simulink model "MDCC"  (R2021b)
settings: Solver=FixedStepDiscrete  StartTime=0.0  StopTime=10.0  FixedStep=0.0001  RelTol=1e-3
model workspace (MATLAB code in the model file):
  | cmdLim = Simulink.Parameter;
  | cmdLim.Value = 15;
  | cmdLim.Description = 'Limit for controlling the maximum surface command angle.';
  | cmdLim.Min = 0;
  | cmdLim.Max = 90;
  | cmdLim.DocUnits = 'deg';
  | 
  | dispGain = Simulink.Parameter;
  | dispGain.Value = 0.75;
  | dispGain.Description = 'Gain applied to the displacement error.';
  | dispGain.Min = 0;
  | dispGain.Max = [];
  | dispGain.DocUnits = 'deg/sec/deg';
  | 
  | dispLim = Simulink.Parameter;
  | dispLim.Value = 30;
  | dispLim.Description = 'Limit for controlling the maximum commanded angle.';
  | dispLim.Min = 0;
  | dispLim.Max = 180;
  | dispLim.DocUnits = 'deg';
  | 
  | intGain = Simulink.Parameter;
  | intGain.Value = 0.5;
  | intGain.Description = 'Gain applied to the integral error.';
  | intGain.Min = 0;
  | intGain.Max = [];
  | intGain.DocUnits = 'deg/sec/deg/sec';
  | 
  | intLim = Simulink.Parameter;
  | intLim.Value = 5;
  | intLim.Description = 'Limit for controlling the maximum commanded angle.';
  | intLim.Min = 0;
  | intLim.Max = 90;
  | intLim.DocUnits = 'deg';
  | 
  | rateGain = Simulink.Parameter;
  | rateGain.Value = 2;
  | rateGain.Description = 'Gain applied to the rate error.';
  | rateGain.Min = 0;
  | rateGain.Max = [];
  | rateGain.DocUnits = 'deg/deg/sec';
  | 
  | rateLim = Simulink.Parameter;
  | rateLim.Value = 6;
  | rateLim.Description = 'Limit for controlling the maximum commanded angle.';
  | rateLim.Min = 0;
  | rateLim.Max = 180;
  | rateLim.DocUnits = 'deg/sec';
  | 
  | hdgGain = Simulink.Parameter;
  | hdgGain.Value = 0.015;
values from neighbouring files (symbols this model uses):
  KfDeadCompen_SetDeltaTime_us = myPackage.Parameter    [DeadCompen.m]
  Ts = 5E-6    (= 5e-06)    [iPMSM_data.m]
  VbDeadComp_SwtUseIsttrDes_flg = myPackage.Parameter    [DeadCompen.m]
  VfDeadCompen_ISttrDdeThdSwt_A = myPackage.Parameter    [DeadCompen.m]
  VfDeadCompen_ISttrIgbtThdSwt_A = myPackage.Parameter    [DeadCompen.m]
  VfDeadCompen_rDdeISttrHi_R = myPackage.Parameter    [DeadCompen.m]
  VfDeadCompen_rDdeISttrLo_R = myPackage.Parameter    [DeadCompen.m]
  VfDeadCompen_rIgbtISttrHi_R = myPackage.Parameter    [DeadCompen.m]
  VfDeadCompen_rIgbtISttrLo_R = myPackage.Parameter    [DeadCompen.m]
  VfDeadCompen_uDdeISttrHi_V = myPackage.Parameter    [DeadCompen.m]
  VfDeadCompen_uDdeISttrLo_V = myPackage.Parameter    [DeadCompen.m]
  VfDeadCompen_uIgbtISttrHi_V = myPackage.Parameter    [DeadCompen.m]
  VfDeadCompen_uIgbtISttrLo_V = myPackage.Parameter    [DeadCompen.m]
undefined symbols (not defined in the file or in its folder): CosTable12bit_Y, GLBCal_GLBCal_Kf_DCLinkOverVolErrThd_V, GLBCal_GLBCal_Kf_DCLinkUnderVolErrThd_V, GLBCal_GLBCal_Kf_EquiLd_NULL, GLBCal_GLBCal_Kf_EquiLq_NULL, GLBCal_GLBCal_Kf_MotorRatedSpeed_rpm, GLBCal_GLBCal_Kf_MotorSpeedHysteresis_Coef, GLBCal_Ke_MotorPolePairsNum_NULL, IoHwAbOpArg_PwmDutyCyclePhU_NULL, IoHwAbOpArg_PwmDutyCyclePhV_NULL, IoHwAbOpArg_PwmDutyCyclePhW_NULL, IoHwAbOpArg_PwmOutputEn, KbMDCC_DeadTimeCompEn_flg, KbMDCC_MCF_flgHarmInIsdqTab11ZR_flg, KbMDCC_MCF_flgHarmInIsdqTab13ZR_flg, KbMDCC_MCF_flgHarmInIsdqTab5ZR_flg, KbMDCC_MCF_flgHarmInIsdqTab7ZR_flg, KbMDCC_MCF_flgHarmInject_flg, KbMDCC_SetEAngleEn_flg, KbMDCC_UdUqFwOmit_flg, KfDeadCompen_CpPeriodTimesT_NULL, KfMDCC_ActiveDischargeIdCurVal_A, KfMDCC_ActiveDischargeIqCurVal_A, KfMDCC_DCLinkVolRate_coef, KfMDCC_DebugEAngleInit_rad, KfMDCC_DebugUalphaVolCmd_V, KfMDCC_DebugUbetaVolCmd_V, KfMDCC_DebugUdCmd_V, KfMDCC_DebugUqCmd_V, KfMDCC_DebugUsCmd_V, KfMDCC_DebugUsRate_V, KfMDCC_IMCResp_NULL, KfMDCC_IMCStab_NULL, KfMDCC_InvParkCpPeriodTimesT_NULL, KfMDCC_MCF_CircAge_NULL, KfMDCC_MCF_flgUse11Harm_flg, KfMDCC_MCF_flgUse13Harm_flg, KfMDCC_MCF_flgUse5Harm_flg, KfMDCC_MCF_flgUse7Harm_flg, KfMDCC_MCF_Harm1113FLParamSpeedThrd_rads, KfMDCC_MCF_Harm57FLParamSpeedThrd_rads, KfMDCC_MCF_HarmcofFltN_NULL, KfMDCC_MCF_HarmCpnAg_NULL, KfMDCC_MCF_HarmfLParaHigh_coef, KfMDCC_MCF_HarmfLParaLow_coef, KfMDCC_MCF_HarmIn1113ZRY_Trq_Nm, KfMDCC_MCF_HarmIn11_SpdLimHigh_rads, KfMDCC_MCF_HarmIn11_SpdLimLow_rads, KfMDCC_MCF_HarmIn11ZRY_Isd_A, KfMDCC_MCF_HarmIn11ZRY_Isq_A, KfMDCC_MCF_HarmIn13_SpdLimHigh_rads, KfMDCC_MCF_HarmIn13_SpdLimLow_rads, KfMDCC_MCF_HarmIn13ZRY_Isd_A, KfMDCC_MCF_HarmIn13ZRY_Isq_A, KfMDCC_MCF_HarmIn57ZRY_Trq_Nm, KfMDCC_MCF_HarmIn5_SpdLimHigh_rads, KfMDCC_MCF_HarmIn5_SpdLimLow_rads, KfMDCC_MCF_HarmIn5ZRY_Isd_A, KfMDCC_MCF_HarmIn5ZRY_Isq_A, KfMDCC_MCF_HarmIn7_SpdLimHigh_rads ... (+47)
libraries: simulink x40, PMSM_Library x3, mcbcontrolslib x1
(part 2 of 8)

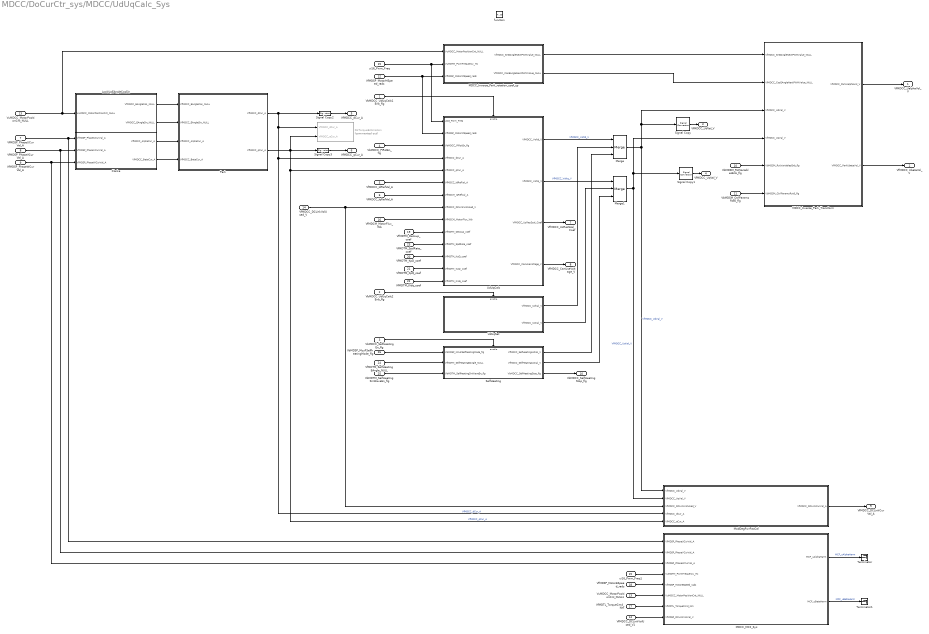
== system MDCC/DoCurCtr_sys/MDCC/UdUqCalc_Sys ==
  VbMDCC_UdUqCalc1Enb_flg : Inport
  VbMDCC_UdUqCalc2Enb_flg : Inport  Port=2
  VbMDCC_SelfHeatingEn_flg : Inport  Port=3
  VbMDCC_PIRstEn_flg : Inport  Port=4
  VfMDCC_IdRefVal_A : Inport  Port=5
  VfMDCC_IqRefVal_A : Inport  Port=6
  VfMDSP_PhaseUCurVal_A : Inport  Port=7
  VfMDSP_PhaseVCurVal_A : Inport  Port=8
  VfMDSP_PhaseWCurVal_A : Inport  Port=9
  VbMDSM_RstVariablesEnb_flg : Inport  Port=10
  VbMDSM_CtrlParamsRst0_flg : Inport  Port=11
  VfMDSP_MotorMSpeed_rads : Inport  Port=12
  VuMDCC_MotorPositionCnt_NULL : Inport  Port=13  OutMin=[0]  OutMax=[4095]
  VfMDCC_DCLinkVolUsed_V : Inport  Port=14
  ui16_Pwm_Freq : Inport  Port=15
  VfMDCM_MotorFlux_Wb : Inport  Port=16
  VfMDTL_TorqueCmd_Nm : Inport  Port=17
  VfMDSP_MotorESpeed_rads : Inport  Port=18
  VfMDTM_Decoup_coef : Inport  Port=19
  VfMDTM_KpD_coef : Inport  Port=20
  VfMDTM_KpQ_coef : Inport  Port=21
  VfMDTM_Kidq_coef : Inport  Port=22
  VfMDTM_SpdRate_coef : Inport  Port=23
  VfMDTM_SelfHeatingEAngle_NULL : Inport  Port=24
  VbMDTM_SelfHeatingSinWaveEn_flg : Inport  Port=25
  VbMDSP_McuFSelfheatingMode_flg : Inport  Port=26
  function : TriggerPort  TriggerType=function-call  VariantControl=Variant  StatesWhenEnabling=reset
      settings: AttributesFormatString=%<StatesWhenEnabling>
  Clarke : Subsystem  TreatAsAtomicUnit=on  RTWFcnName=vPwm_MDCC_Clarke  RTWFileName=MDCC
      settings: RTWSystemCode=Nonreusable function  RTWFcnNameOpts=User specified
  DoTorqueEstimation : Subsystem  Commented=on  TreatAsAtomicUnit=on  RTWFcnName=DoTorqueEstimation  RTWFileName=MDCC
      settings: RTWSystemCode=Nonreusable function  RTWFcnNameOpts=User specified
  LookUpEAngleCosSin : Subsystem  TreatAsAtomicUnit=on  RTWFcnName=vPwm_MDCC_LookUpEAngleCosSin  RTWFileName=MDCC
      settings: RTWSystemCode=Nonreusable function  RTWFcnNameOpts=User specified
  MDCC_Inverse_Park_Transform : Subsystem  TreatAsAtomicUnit=on  RTWFcnName=MDCC_Inverse_Park_Transform  RTWFileName=MDCC
      settings: RTWSystemCode=Nonreusable function  RTWFcnNameOpts=User specified  FunctionWithSeparateData=on
  MDCC_Inverse_Park_rotation_coef_cp : Subsystem  TreatAsAtomicUnit=on  RTWFcnName=MDCC_Inverse_Park_rotation_coef_cp  RTWFileName=MDCC
      settings: RTWSystemCode=Nonreusable function  RTWFcnNameOpts=User specified  FunctionWithSeparateData=on
  MDCC_MCF_Sys : Subsystem
      settings: RTWSystemCode=Nonreusable function  RTWFcnNameOpts=Use subsystem name
  Merge : Merge  Inputs=3
  Merge1 : Merge  Inputs=3
  ModDegPwrFacCal : Subsystem  TreatAsAtomicUnit=on  RTWFcnName=ModDegPwrFacCal  RTWFileName=MDCC
      settings: RTWSystemCode=Nonreusable function  RTWFcnNameOpts=User specified
  Park : Subsystem  TreatAsAtomicUnit=on  RTWFcnName=vPwm_MDCC_Park  RTWFileName=MDCC
      settings: RTWSystemCode=Nonreusable function  RTWFcnNameOpts=User specified
  SelfHeating : Subsystem
  Signal Copy{,1..3} (4 alike) : SignalConversion  OverrideOpt=off
  Terminator : Terminator
  Terminator1 : Terminator
  UdUqCalc : Subsystem  TreatAsAtomicUnit=on  RTWFcnName=MDCC_UdUqCalc
      settings: RTWSystemCode=Nonreusable function  RTWFcnNameOpts=User specified  FunctionWithSeparateData=on
  UdUqSet : Subsystem  RTWFcnName=MDCC_Debug_UdUqSet
      settings: RTWSystemCode=Nonreusable function  RTWFcnNameOpts=User specified
  VfMDCC_DCLinkVolUsed_V1 : InportShadow  Port=14
  VuMDCC_MotorPositionCnt_NULL1 : InportShadow  Port=13  OutMin=[0]  OutMax=[4095]
  ui16_Pwm_Freq1 : InportShadow  Port=15
  VfMDCC_UalphaVol_V : Outport
  VfMDCC_UbetaVol_V : Outport  Port=2
  VfMDCC_UdVal_V : Outport  Port=3
  VfMDCC_UqVal_V : Outport  Port=4
  VfMDCC_dCur_A : Outport  Port=5
  VfMDCC_qCur_A : Outport  Port=6
  VfMDCC_UsResScal_Coef : Outport  Port=7
  VfMDCC_CanUseVoltage_V : Outport  Port=8
  VfMDCC_DCLinkCurVal_A : Outport  Port=9
  VbMDCC_SelfHeatingStop_flg : Outport  Port=10
  wires:
  VfMDCC_IdRefVal_A/1 -> UdUqCalc/6(VfMDCC_IdRefVal_A)
  VfMDCC_IqRefVal_A/1 -> UdUqCalc/7(VfMDCM_IqRefVal_A)
  VfMDSP_MotorMSpeed_rads/1 -> UdUqCalc/2(VfMDSP_MotorMSpeed_rads), MDCC_Inverse_Park_rotation_coef_cp/3(VfMDSP_MotorMSpeed_rads)
  ui16_Pwm_Freq/1 -> UdUqCalc/1(ui16_Pwm_Freq), MDCC_Inverse_Park_rotation_coef_cp/2(VuMDTM_PwmFrequency_Hz)
  VbMDCC_UdUqCalc1Enb_flg/1 -> UdUqCalc/Enable
  VbMDCC_UdUqCalc2Enb_flg/1 -> UdUqSet/Enable
  VbMDSM_RstVariablesEnb_flg/1 -> MDCC_Inverse_Park_Transform/5(VbMDSM_RstVariablesEnb_flg)
  VbMDSM_CtrlParamsRst0_flg/1 -> MDCC_Inverse_Park_Transform/6(VbMDSM_CtrlParamsRst0_flg)
  VuMDCC_MotorPositionCnt_NULL/1 -> MDCC_Inverse_Park_rotation_coef_cp/1(VuMDCC_MotorPositionCnt_NULL), LookUpEAngleCosSin/1(VuMDCC_MotorPositionCnt_NULL)
  LookUpEAngleCosSin/1(VfMDCC_EAngleCos_NULL) -> Park/1(VfMDCC_EAngleCos_NULL)
  Clarke/1(VfMDCC_AlphaCur_A) -> Park/3(VfMDCC_AlphaCur_A)
  Clarke/2(VfMDCC_BetaCur_A) -> Park/4(VfMDCC_BetaCur_A)
  Park/2(VfMDCC_qCur_A) -> DoTorqueEstimation/2(VfMDCC_qCur_A), Signal Copy3/1, ModDegPwrFacCal/5(VfMDCC_qCur_A), UdUqCalc/5(VfMDCC_qCur_A)  "VfMDCC_qCur_A"
  Park/1(VfMDCC_dCur_A) -> ModDegPwrFacCal/4(VfMDCC_dCur_A), UdUqCalc/4(VfMDCC_dCur_A), DoTorqueEstimation/1(VfMDCC_dCur_A), Signal Copy2/1  "VfMDCC_dCur_A"
  LookUpEAngleCosSin/2(VfMDCC_EAngleSin_NULL) -> Park/2(VfMDCC_EAngleSin_NULL)
  VfMDSP_PhaseUCurVal_A/1 -> MDCC_MCF_Sys/1(VfMDSP_PhaseUCurVal_A), Clarke/1(VfMDSP_PhaseUCurVal_A)
  VfMDSP_PhaseVCurVal_A/1 -> MDCC_MCF_Sys/2(VfMDSP_PhaseVCurVal_A), Clarke/2(VfMDSP_PhaseVCurVal_A)
  VfMDSP_PhaseWCurVal_A/1 -> Clarke/3(VfMDSP_PhaseWCurVal_A), MDCC_MCF_Sys/3(VfMDSP_PhaseWCurVal_A)
  MDCC_Inverse_Park_rotation_coef_cp/1(VfMDCC_SinEAngleNextPWMValue_NULL) -> MDCC_Inverse_Park_Transform/1(VfMDCC_SinEAngleNextPWMValue_NULL)
  MDCC_Inverse_Park_rotation_coef_cp/2(VfMDCC_CosEAngleNextPWMValue_NULL) -> MDCC_Inverse_Park_Transform/2(VfMDCC_CosEAngleNextPWMValue_NULL)
  VfMDCC_DCLinkVolUsed_V/1 -> UdUqCalc/8(VfMDCC_DCLinkVolUsed_V), ModDegPwrFacCal/3(VfMDCC_DCLinkVolUsed_V)
  Merge/1 -> ModDegPwrFacCal/1(VfMDCC_UdVal_V), MDCC_Inverse_Park_Transform/3(VfMDCC_UdVal_V), Signal Copy/1  "VfMDCC_UdVal_V"
  Merge1/1 -> MDCC_Inverse_Park_Transform/4(VfMDCC_UqVal_V), Signal Copy1/1, ModDegPwrFacCal/2(VfMDCC_UqVal_V)  "VfMDCC_UqVal_V"
  VfMDCM_MotorFlux_Wb/1 -> UdUqCalc/9(VfMDCM_MotorFlux_Wb)
  UdUqCalc/3(VfMDCC_UsResScal_Coef) -> VfMDCC_UsResScal_Coef/1
  UdUqCalc/4(VfMDCC_CanUseVoltage_V) -> VfMDCC_CanUseVoltage_V/1
  VbMDCC_PIRstEn_flg/1 -> UdUqCalc/3(VbMDCC_PIRstEn_flg)
  Signal Copy/1 -> VfMDCC_UdVal_V/1
  Signal Copy1/1 -> VfMDCC_UqVal_V/1
  UdUqCalc/1(VfMDCC_Voltd_V) -> Merge/1  "VfMDCC_Voltd_V"
  UdUqSet/1(VfMDCC_UdVal_V) -> Merge/2
  UdUqCalc/2(VfMDCC_Voltq_V) -> Merge1/1  "VfMDCC_Voltq_V"
  UdUqSet/2(VfMDCC_UqVal_V) -> Merge1/2
  VfMDSP_MotorESpeed_rads/1 -> MDCC_MCF_Sys/5(VfMDSP_MotorESpeed_rads)
  VfMDTL_TorqueCmd_Nm/1 -> MDCC_MCF_Sys/7(VfMDTL_TorqueCmd_Nm)
  ui16_Pwm_Freq1/1 -> MDCC_MCF_Sys/4(VuMDTM_PwmFrequency_Hz)
  VuMDCC_MotorPositionCnt_NULL1/1 -> MDCC_MCF_Sys/6(VuMDCC_MotorPositionCnt_NULL)
  VfMDCC_DCLinkVolUsed_V1/1 -> MDCC_MCF_Sys/8(VfMDSP_DCLinkVolVal_V)
  MDCC_Inverse_Park_Transform/1(VfMDCC_ParkUalphaVol_V) -> VfMDCC_UalphaVol_V/1
  MDCC_Inverse_Park_Transform/2(VfMDCC_ParkUbetaVol_V) -> VfMDCC_UbetaVol_V/1
  ModDegPwrFacCal/1(VfMDCC_DCLinkCurVal_A) -> VfMDCC_DCLinkCurVal_A/1
  VfMDTM_SpdRate_coef/1 -> UdUqCalc/11(VfMDTM_SpdRate_coef)
  VfMDTM_KpD_coef/1 -> UdUqCalc/12(VfMDTM_KpD_coef)
  VfMDTM_Kidq_coef/1 -> UdUqCalc/14(VfMDTM_Kidq_coef)
  VfMDTM_KpQ_coef/1 -> UdUqCalc/13(VfMDTM_KpQ_coef)
  VfMDTM_Decoup_coef/1 -> UdUqCalc/10(VfMDTM_Decoup_coef)
  Signal Copy2/1 -> VfMDCC_dCur_A/1
  Signal Copy3/1 -> VfMDCC_qCur_A/1
  VfMDTM_SelfHeatingEAngle_NULL/1 -> SelfHeating/2(VfMDTM_SelfHeatingEAngle_NULL)
  VbMDCC_SelfHeatingEn_flg/1 -> SelfHeating/Enable
  SelfHeating/1(VfMDCC_SelfHeatingUdVal_V) -> Merge/3
  SelfHeating/2(VfMDCC_SelfHeatingUqVal_V) -> Merge1/3
  VbMDTM_SelfHeatingSinWaveEn_flg/1 -> SelfHeating/3(VbMDTM_SelfHeatingSinWaveEn_flg)
  SelfHeating/3(VbMDCC_SelfHeatingStop_flg) -> VbMDCC_SelfHeatingStop_flg/1
  VbMDSP_McuFSelfheatingMode_flg/1 -> SelfHeating/1(VbMDSP_McuFSelfheatingMode_flg)
  MDCC_MCF_Sys/1(MCF_uAlphaHarm) -> Terminator/1  "MCF_uAlphaHarm"
  MDCC_MCF_Sys/2(MCF_uBetaHarm) -> Terminator1/1  "MCF_uBetaHarm"

== system MDCC/DoCurCtr_sys/MDCC/IrmsCalc_Sys/Enabled Subsystem ==
  A2_Rms : Inport
  B2_Rms : Inport  Port=2
  C2_Rms : Inport  Port=3
  Enable : EnablePort
  Gain1 : Gain  Gain=10
  Gain2 : Gain  Gain=10
  Gain3 : Gain  Gain=10
  Sqrt : Sqrt  SaturateOnIntegerOverflow=on
  Sqrt1 : Sqrt  SaturateOnIntegerOverflow=on
  Sqrt2 : Sqrt  SaturateOnIntegerOverflow=on
  A_Rms_Out : Outport
  B_Rms_Out : Outport  Port=2
  C_Rms_Out : Outport  Port=3
  wires:
  A2_Rms/1 -> Gain1/1
  Sqrt/1 -> A_Rms_Out/1
  B2_Rms/1 -> Gain2/1
  C2_Rms/1 -> Gain3/1
  Gain1/1 -> Sqrt/1
  Sqrt1/1 -> B_Rms_Out/1
  Gain2/1 -> Sqrt1/1
  Gain3/1 -> Sqrt2/1
  Sqrt2/1 -> C_Rms_Out/1

== system MDCC/DoCurCtr_sys/MDCC/IrmsCalc_Sys/Subsystem ==
  Add1 : Sum
  Compare To Constant : simulink/Logic and Bit Operations/Compare To Constant  relop=>=  const=1000  OutDataTypeStr=boolean
  Constant : Constant
  Constant1 : Constant  Value=0  OutDataTypeStr=uint16
  Delay : Delay  DelayLength=1
  Delay1 : Delay  DelayLength=1
  OR : Logic  Operator=OR  AllPortsSameDT=off  OutDataTypeStr=boolean
  Switch : Switch  Criteria=u2 ~= 0
  RmsValueValid : Outport
  Vector : Outport  Port=2
  wires:
  Constant1/1 -> Switch/1
  Compare To Constant/1 -> OR/1, Delay/1, Switch/2
  Switch/1 -> Delay1/1
  Constant/1 -> Add1/1
  Add1/1 -> Compare To Constant/1, Switch/3
  Delay1/1 -> Vector/1, Add1/2
  Delay/1 -> OR/2
  OR/1 -> RmsValueValid/1

== system MDCC/DoCurCtr_sys/MDCC/IrmsCalc_Sys/Subsystem1 ==
  Vector : Inport
  PreArray_A : Inport  Port=2
  PreArray_B : Inport  Port=3
  PreArray_C : Inport  Port=4
  Trigger : TriggerPort  TriggerType=function-call  VariantControl=(inherit)  PortDimensions=1
  Index Vector : MultiPortSwitch  DataPortOrder=Zero-based contiguous  Inputs=1  zeroidx=on
  Index Vector1 : MultiPortSwitch  DataPortOrder=Zero-based contiguous  Inputs=1  zeroidx=on
  Index Vector2 : MultiPortSwitch  DataPortOrder=Zero-based contiguous  Inputs=1  zeroidx=on
  Earliest_Element_A : Outport
  Earliest_Element_B : Outport  Port=2
  Earliest_Element_C : Outport  Port=3
  wires:
  Index Vector/1 -> Earliest_Element_A/1
  Vector/1 -> Index Vector2/1, Index Vector1/1, Index Vector/1
  PreArray_A/1 -> Index Vector/2
  PreArray_C/1 -> Index Vector2/2
  PreArray_B/1 -> Index Vector1/2
  Index Vector1/1 -> Earliest_Element_B/1
  Index Vector2/1 -> Earliest_Element_C/1

== system MDCC/DoCurCtr_sys/MDCC/IrmsCalc_Sys/Subsystem2 ==
  Vector : Inport
  Element_Inlet_A : Inport  Port=2
  Element_Inlet_B : Inport  Port=3
  Element_Inlet_C : Inport  Port=4
  Trigger : TriggerPort  TriggerType=function-call  VariantControl=(inherit)  PortDimensions=1
  Assignment : Assignment  IndexMode=Zero-based  DiagnosticForDimensions=Warning  IndexOptions=Index vector (port)  Indices=1  OutputSizes=1
  Assignment1 : Assignment  IndexMode=Zero-based  DiagnosticForDimensions=Warning  IndexOptions=Index vector (port)  Indices=1  OutputSizes=1
  Assignment2 : Assignment  IndexMode=Zero-based  DiagnosticForDimensions=Warning  IndexOptions=Index vector (port)  Indices=1  OutputSizes=1
  Data Store Read : DataStoreRead  DataStoreName=Array_A  IndexOptions=Index vector (dialog)  Indices=1  OutputSizes=1
  Data Store Read1 : DataStoreRead  DataStoreName=Array_B  IndexOptions=Index vector (dialog)  Indices=1  OutputSizes=1
  Data Store Read2 : DataStoreRead  DataStoreName=Array_C  IndexOptions=Index vector (dialog)  Indices=1  OutputSizes=1
  Data Store Write : DataStoreWrite  DataStoreName=Array_A  IndexOptions=Index vector (dialog)  Indices=1  OutputSizes=1
  Data Store Write1 : DataStoreWrite  DataStoreName=Array_C  IndexOptions=Index vector (dialog)  Indices=1  OutputSizes=1
  Data Store Write2 : DataStoreWrite  DataStoreName=Array_B  IndexOptions=Index vector (dialog)  Indices=1  OutputSizes=1
  wires:
  Data Store Read/1 -> Assignment/1
  Element_Inlet_A/1 -> Assignment/2
  Assignment/1 -> Data Store Write/1
  Vector/1 -> Assignment2/3, Assignment1/3, Assignment/3
  Element_Inlet_B/1 -> Assignment1/2
  Data Store Read1/1 -> Assignment1/1
  Assignment1/1 -> Data Store Write2/1
  Element_Inlet_C/1 -> Assignment2/2
  Data Store Read2/1 -> Assignment2/1
  Assignment2/1 -> Data Store Write1/1

== system MDCC/DoCurCtr_sys/MDCC/IrmsCalc_Sys/Subsystem3 ==
  Earliest_Element_A : Inport
  Element_Inlet_A : Inport  Port=2
  Earliest_Element_B : Inport  Port=3
  Element_Inlet_B : Inport  Port=4
  Earliest_Element_C : Inport  Port=5
  Element_Inlet_C : Inport  Port=6
  Trigger : TriggerPort  TriggerType=function-call  VariantControl=(inherit)  PortDimensions=1
  Subsystem : Subsystem
  Subsystem1 : Subsystem
  Subsystem2 : Subsystem
  A2_Rms : Outport
  B2_Rms : Outport  Port=2
  C2_Rms : Outport  Port=3
  wires:
  Earliest_Element_A/1 -> Subsystem/1(Earliest_Element)
  Element_Inlet_A/1 -> Subsystem/2(Element_Inlet)
  Subsystem/1(Rms) -> A2_Rms/1
  Element_Inlet_B/1 -> Subsystem1/2(Element_Inlet)
  Earliest_Element_B/1 -> Subsystem1/1(Earliest_Element)
  Element_Inlet_C/1 -> Subsystem2/2(Element_Inlet)
  Earliest_Element_C/1 -> Subsystem2/1(Earliest_Element)
  Subsystem1/1(Rms) -> B2_Rms/1
  Subsystem2/1(Rms) -> C2_Rms/1

== system MDCC/DoCurCtr_sys/MDCC/MDCC_Debug_Us/EAngleOL1 ==
  VuMDTM_PwmFrequency_Hz : Inport
  VfMDSP_MotorMSpeed_rads : Inport  Port=2
  Constant : Constant  Value=KbMDCC_SetEAngleEn_flg
  Constant1 : Constant  Value=CosTable12bit_Y
  Constant3 : Constant  Value=SinTable12bit_Y
  Constant4 : Constant  Value=KuMDCC_SetEAngle_Null  OutMin=0  OutMax=360  OutDataTypeStr=single
  Direct Lookup Table (n-D) : LookupNDDirect  NumberOfTableDimensions=1  TableIsInput=on  Table=[4 5 6]  TableMax=[4096]
  Direct Lookup Table (n-D)1 : LookupNDDirect  NumberOfTableDimensions=1  TableIsInput=on  Table=[4 5 6]  TableMax=[4096]
  GLBCal_Ke_MotorPolePairsNum_NULL : Constant  Value=GLBCal_Ke_MotorPolePairsNum_NULL
  Ku_EAngleSet_Caller : FunctionCaller  FunctionPrototype=Vu_AutoEAngle_NULL = Ku_EAngleSet(Kf_SpdCmd_rads,Vu_PwmFrequency_Hz,Ke_MotorPolePairsNum_NULL,Kb_SetEAngleFixValEn_flg,Kf_SetEAngle_Null)  InputArgumentSpecifications=single(0),uint16(0),uint8(0),boolean(0),single(0)  OutputArgumentSpecifications=uint16(0)
  cos : Outport
  sin : Outport  Port=2
  wires:
  Ku_EAngleSet_Caller/1 -> Direct Lookup Table (n-D)1/1, Direct Lookup Table (n-D)/1  "Vu_AutoEAngle_NULL"
  Constant1/1 -> Direct Lookup Table (n-D)/2
  Constant3/1 -> Direct Lookup Table (n-D)1/2
  Direct Lookup Table (n-D)/1 -> cos/1
  Direct Lookup Table (n-D)1/1 -> sin/1
  VfMDSP_MotorMSpeed_rads/1 -> Ku_EAngleSet_Caller/1
  GLBCal_Ke_MotorPolePairsNum_NULL/1 -> Ku_EAngleSet_Caller/3
  VuMDTM_PwmFrequency_Hz/1 -> Ku_EAngleSet_Caller/2
  Constant/1 -> Ku_EAngleSet_Caller/4
  Constant4/1 -> Ku_EAngleSet_Caller/5

== system MDCC/DoCurCtr_sys/MDCC/MDCC_Debug_Us/VolOL ==
  KfMDCC_DebugUsCmd_V : Constant  Value=KfMDCC_DebugUsCmd_V  OutDataTypeStr=single
  KfMDCC_DebugUsRate_V : Constant  Value=KfMDCC_DebugUsRate_V  OutDataTypeStr=single
  Unit Delay : UnitDelay  SampleTime=-1  HasFrameUpgradeWarning=on
  slope : PMSM_Library/slope  SystemSampleTime=-1  VariantActivationTime=update diagram  Latency=0  AutoFrameSizeCalculation=off
  UsSlope : Outport
  wires:
  Unit Delay/1 -> slope/2
  KfMDCC_DebugUsRate_V/1 -> slope/3
  KfMDCC_DebugUsCmd_V/1 -> slope/1
  slope/1 -> Unit Delay/1, UsSlope/1

== system MDCC/DoCurCtr_sys/MDCC/SVM_Calc/DeadComp_Sys ==
  U_Phase_Dyc : Inport
  V_Phase_Dyc : Inport  Port=2
  W_Phase_Dyc : Inport  Port=3
  IsdDes_A : Inport  Port=4
  IsqDes_A : Inport  Port=5
  IsdFb_A : Inport  Port=6
  IsqFb_A : Inport  Port=7
  agPreRtrEl : Inport  Port=8
  PwmFreq_Hz : Inport  Port=9
  uDcLink : Inport  Port=10
  VfMDSP_MotorMSpeed_rads : Inport  Port=11
  Enable : EnablePort
  Constant1 : Constant  Value=GLBCal_Ke_MotorPolePairsNum_NULL
  Constant3 : Constant  Value=single(1/(2*pi))
  DeadCur_Calc : Subsystem  TreatAsAtomicUnit=on
      settings: RTWSystemCode=Nonreusable function
  DeadDuty_Calc : Subsystem
  DeadTime_Calc : Subsystem
  Product : Product  Inputs=3
  PwmFreq_Hz1 : InportShadow  Port=9
  VfMDCC_PWMDutyUDeadCompFINAL_NULL : Outport
  VfMDCC_PWMDutyVDeadCompFINAL_NULL : Outport  Port=2
  VfMDCC_PWMDutyWDeadCompFINAL_NULL : Outport  Port=3
  wires:
  IsdFb_A/1 -> DeadCur_Calc/3(IsdFb_A)
  IsqFb_A/1 -> DeadCur_Calc/4(IsqFb_A)
  Product/1 -> DeadCur_Calc/5(FrqRtrEl_Hz)
  agPreRtrEl/1 -> DeadCur_Calc/6(agPreRtrEl)
  DeadCur_Calc/4(CntSctrIs) -> DeadDuty_Calc/2(CntSctrIs)
  IsqDes_A/1 -> DeadCur_Calc/2(IsqDes_A)
  IsdDes_A/1 -> DeadCur_Calc/1(IsdDes_A)
  U_Phase_Dyc/1 -> DeadTime_Calc/1(U_Phase_Dyc)  "DutyPhaseU"
  DeadCur_Calc/1(iaPre) -> DeadTime_Calc/4(iPhase_U)
  V_Phase_Dyc/1 -> DeadTime_Calc/2(V_Phase_Dyc)  "DutyPhaseV"
  DeadCur_Calc/2(ibPre) -> DeadTime_Calc/5(iPhase_V)
  DeadCur_Calc/3(icPre) -> DeadTime_Calc/6(iPhase_W)
  W_Phase_Dyc/1 -> DeadTime_Calc/3(W_Phase_Dyc)  "DutyPhaseW"
  PwmFreq_Hz/1 -> DeadCur_Calc/7(PwmFreq_Hz)
  uDcLink/1 -> DeadTime_Calc/7(uDcLink)
  Constant1/1 -> Product/2
  VfMDSP_MotorMSpeed_rads/1 -> Product/1
  Constant3/1 -> Product/3
  DeadDuty_Calc/1(VfMDSA_DeadCompPwmDutyCyclePhaseU_NULL) -> VfMDCC_PWMDutyUDeadCompFINAL_NULL/1
  DeadDuty_Calc/2(VfMDSA_DeadCompPwmDutyCyclePhaseV_NULL) -> VfMDCC_PWMDutyVDeadCompFINAL_NULL/1
  DeadDuty_Calc/3(VfMDSA_DeadCompPwmDutyCyclePhaseW_NULL) -> VfMDCC_PWMDutyWDeadCompFINAL_NULL/1
  PwmFreq_Hz1/1 -> DeadTime_Calc/8(PwmFreq_Hz)
  DeadTime_Calc/1(Bus_DutyCompensate) -> DeadDuty_Calc/1(Bus_DutyCompensate)

== system MDCC/DoCurCtr_sys/MDCC/SVM_Calc/MDSA ==
  VfMDCC_Ualpha_V : Inport
  VfMDCC_Ubeta_V : Inport  Port=2
  VfMDCC_DCLinkVolUsed_V : Inport  Port=3
  VuMDTM_PwmFrequency_Hz : Inport  Port=4
  Constant : Constant  Value=single(1)
  Divide : Product  Inputs=*/
  Divide1 : Product  Inputs=*/
  Divide2 : Product  Inputs=*/
  SVM_PU : Subsystem  TreatAsAtomicUnit=on  RTWFcnName=SVPWM_Calc
      settings: RTWSystemCode=Nonreusable function  RTWFcnNameOpts=User specified
  SVPWM : Subsystem  Commented=on  AncestorBlock=SVPWM/SVPWM  TreatAsAtomicUnit=on  RTWFcnName=SVPWM  RTWFileName=SVPWM
      settings: RTWFcnNameOpts=User specified
  VfMDSA_PwmDutyCyclePhaseU_NULL : Outport  OutMin=0  OutMax=1
  VfMDSA_PwmDutyCyclePhaseV_NULL : Outport  Port=2  OutMin=0  OutMax=1
  VfMDSA_PwmDutyCyclePhaseW_NULL : Outport  Port=3  OutMin=0  OutMax=1
  wires:
  VfMDCC_Ualpha_V/1 -> SVPWM/1(Ualpha_V), Divide1/1
  VfMDCC_Ubeta_V/1 -> Divide2/1, SVPWM/2(Ubeta_V)
  Constant/1 -> Divide/1
  Divide/1 -> SVPWM/3(Ts)  "VfMDSA_TsUsedInSVPWM_s"
  VuMDTM_PwmFrequency_Hz/1 -> Divide/2
  VfMDCC_DCLinkVolUsed_V/1 -> SVPWM/4(Vdc), Divide1/2, Divide2/2
  Divide1/1 -> SVM_PU/1(Ualpha)
  Divide2/1 -> SVM_PU/2(Ubeta)
  SVM_PU/1(VfMDSA_PwmDutyCyclePhaseU_NULL) -> VfMDSA_PwmDutyCyclePhaseU_NULL/1
  SVM_PU/2(VfMDSA_PwmDutyCyclePhaseV_NULL) -> VfMDSA_PwmDutyCyclePhaseV_NULL/1
  SVM_PU/3(VfMDSA_PwmDutyCyclePhaseW_NULL) -> VfMDSA_PwmDutyCyclePhaseW_NULL/1

== system MDCC/DoCurCtr_sys/MDCC/Simulink Function/Enabled Subsystem ==
  Kf_SetEAngle_Null : Inport
  Enable : EnablePort
  pi_180 : Gain  Gain=pi/180  OutDataTypeStr=single
  Vf_AutoEAngle_NULL : Outport
  wires:
  Kf_SetEAngle_Null/1 -> pi_180/1
  pi_180/1 -> Vf_AutoEAngle_NULL/1

== system MDCC/DoCurCtr_sys/MDCC/Simulink Function/Subsystem ==
  Ke_MotorPolePairsNum_NULL : Inport
  Kf_SpdCmd_rads : Inport  Port=2
  Vu_PwmFrequency_Hz : Inport  Port=3
  Enable : EnablePort
  Constant2 : Constant  Value=2*pi  OutDataTypeStr=single
  Divide : Product  Inputs=*/
  Divide1 : Product  Inputs=**
  If Action Subsystem : Subsystem  TreatAsAtomicUnit=on
  If Action Subsystem1 : Subsystem  TreatAsAtomicUnit=on
  If Action Subsystem2 : Subsystem  TreatAsAtomicUnit=on
  If1 : If  NumInputs=2  IfExpression=u1 >= u2  ElseIfExpressions=u1 <0
  KfMDCC_DebugEAngleInit_rad : Constant  Value=KfMDCC_DebugEAngleInit_rad  OutDataTypeStr=single
  Merge : Merge  Inputs=3
  Resettable Delay : Delay  DelayLength=1  InitialConditionSource=Input port
      settings: InputPortMap=u0,p4
  Sum4 : Sum  Inputs=|++
  Vf_AutoEAngle_NULL : Outport
  wires:
  Resettable Delay/1 -> Sum4/2
  If Action Subsystem/1(Out1) -> Merge/1
  Sum4/1 -> If1/1, If Action Subsystem/1(In1), If Action Subsystem1/1(In1), If Action Subsystem2/1(In1)
  If1/1 -> If Action Subsystem/Action
  Divide/1 -> Sum4/1
  Divide1/1 -> Divide/1
  If Action Subsystem2/1(Out1) -> Merge/3
  Constant2/1 -> If1/2
  If1/2 -> If Action Subsystem1/Action
  KfMDCC_DebugEAngleInit_rad/1 -> Resettable Delay/2
  Kf_SpdCmd_rads/1 -> Divide1/2
  If Action Subsystem1/1(Out1) -> Merge/2
  If1/3 -> If Action Subsystem2/Action
  Ke_MotorPolePairsNum_NULL/1 -> Divide1/1
  Vu_PwmFrequency_Hz/1 -> Divide/2
  Merge/1 -> Vf_AutoEAngle_NULL/1, Resettable Delay/1

== system MDCC/DoCurCtr_sys/MDCC/UdUqCalc_Sys/Clarke ==
  VfMDSP_PhaseUCurVal_A : Inport
  VfMDSP_PhaseVCurVal_A : Inport  Port=2
  VfMDSP_PhaseWCurVal_A : Inport  Port=3
  Constant : Constant  Value=0.57735  OutDataTypeStr=single
  Data Type Conversion : DataTypeConversion  OutDataTypeStr=single
  Product : Product
  Subtract : Sum  Inputs=+-
  VfMDCC_AlphaCur_A : Outport
  VfMDCC_BetaCur_A : Outport  Port=2
  wires:
  Data Type Conversion/1 -> VfMDCC_AlphaCur_A/1  "VfMDCC_AlphaCur_A"
  Product/1 -> VfMDCC_BetaCur_A/1  "VfMDCC_BetaCur_A"
  Constant/1 -> Product/2
  Subtract/1 -> Product/1
  VfMDSP_PhaseWCurVal_A/1 -> Subtract/2
  VfMDSP_PhaseVCurVal_A/1 -> Subtract/1
  VfMDSP_PhaseUCurVal_A/1 -> Data Type Conversion/1

== system MDCC/DoCurCtr_sys/MDCC/UdUqCalc_Sys/DoTorqueEstimation ==
  VfMDCC_dCur_A : Inport
  VfMDCC_qCur_A : Inport  Port=2
  Constant : Constant  Value=KfMDCC_TqEsFltFactorNow_NULL
  Constant2 : Constant  Value=boolean(1)
  Delay : Delay  DelayLength=1
  Interpolation Using Prelookup Id : Interpolation_n-D  Table=TqArrayForTqEs  ExtrapMethod=Clip  RemoveProtectionIndex=on  InternalRulePriority=Speed
  One_Order_LP : PMSM_Library/One_Order_LP  SystemSampleTime=-1  VariantActivationTime=update diagram  Latency=0  AutoFrameSizeCalculation=off
  Prelookup_Wn : PreLookup  BreakpointsData=IqArrayForTqEs  IndexSearchMethod=Evenly spaced points  ExtrapMethod=Linear
  Prelookup_Wn1 : PreLookup  BreakpointsData=IdArrayForTqEs  IndexSearchMethod=Evenly spaced points  ExtrapMethod=Linear
  Terminator : Terminator
  wires:
  Delay/1 -> One_Order_LP/3
  Interpolation Using Prelookup Id/1 -> One_Order_LP/1
  Prelookup_Wn1/1 -> Interpolation Using Prelookup Id/3
  Prelookup_Wn1/2 -> Interpolation Using Prelookup Id/4
  Prelookup_Wn/2 -> Interpolation Using Prelookup Id/2
  Prelookup_Wn/1 -> Interpolation Using Prelookup Id/1
  VfMDCC_qCur_A/1 -> Prelookup_Wn/1
  VfMDCC_dCur_A/1 -> Prelookup_Wn1/1
  One_Order_LP/1 -> Delay/1, Terminator/1  "VfMDCC_TqEstimated_Nm"
  Constant/1 -> One_Order_LP/2
  Constant2/1 -> One_Order_LP/Enable

== system MDCC/DoCurCtr_sys/MDCC/UdUqCalc_Sys/LookUpEAngleCosSin ==
  VuMDCC_MotorPositionCnt_NULL : Inport  OutMin=[0]  OutMax=[4095]
  Constant2 : Constant  Value=CosTable12bit_Y
  Constant3 : Constant  Value=SinTable12bit_Y
  Direct Lookup Table (n-D) : LookupNDDirect  NumberOfTableDimensions=1  TableIsInput=on  Table=[4 5 6]  TableMax=[4096]
  Direct Lookup Table (n-D)1 : LookupNDDirect  NumberOfTableDimensions=1  TableIsInput=on  Table=[4 5 6]  TableMax=[4096]
  VfMDCC_EAngleCos_NULL : Outport
  VfMDCC_EAngleSin_NULL : Outport  Port=2
  wires:
  VuMDCC_MotorPositionCnt_NULL/1 -> Direct Lookup Table (n-D)/1, Direct Lookup Table (n-D)1/1
  Direct Lookup Table (n-D)/1 -> VfMDCC_EAngleCos_NULL/1  "VfMDCC_EAngleCos_NULL"
  Direct Lookup Table (n-D)1/1 -> VfMDCC_EAngleSin_NULL/1  "VfMDCC_EAngleSin_NULL"
  Constant2/1 -> Direct Lookup Table (n-D)/2
  Constant3/1 -> Direct Lookup Table (n-D)1/2

== system MDCC/DoCurCtr_sys/MDCC/UdUqCalc_Sys/MDCC_Inverse_Park_Transform ==
  VfMDCC_SinEAngleNextPWMValue_NULL : Inport
  VfMDCC_CosEAngleNextPWMValue_NULL : Inport  Port=2
  VfMDCC_UdVal_V : Inport  Port=3
  VfMDCC_UqVal_V : Inport  Port=4
  VbMDSM_RstVariablesEnb_flg : Inport  Port=5
  VbMDSM_CtrlParamsRst0_flg : Inport  Port=6
  Constant : Constant  Value=single(0)
  Constant1 : Constant  Value=single(0)
  Do_Inverse_Park_Transform : Subsystem  TreatAsAtomicUnit=on  RTWFcnName=vIntp_PWMFOC_InverseParkTrans  RTWFileName=Transform
      settings: RTWSystemCode=Nonreusable function  RTWFcnNameOpts=User specified
  Logical Operator : Logic  Operator=OR  AllPortsSameDT=off  OutDataTypeStr=boolean
  Switch1 : Switch  Criteria=u2 ~= 0
  Switch2 : Switch  Criteria=u2 ~= 0
  VfMDCC_ParkUalphaVol_V : Outport
  VfMDCC_ParkUbetaVol_V : Outport  Port=2
  wires:
  Constant1/1 -> Switch2/1
  Switch1/1 -> VfMDCC_ParkUalphaVol_V/1
  Switch2/1 -> VfMDCC_ParkUbetaVol_V/1
  Constant/1 -> Switch1/1
  Logical Operator/1 -> Switch2/2, Switch1/2
  Do_Inverse_Park_Transform/2(VfMDCC_VolCmd_beta_V) -> Switch2/3
  Do_Inverse_Park_Transform/1(VfMDCC_VolCmd_alpha_V) -> Switch1/3
  VbMDSM_RstVariablesEnb_flg/1 -> Logical Operator/1
  VbMDSM_CtrlParamsRst0_flg/1 -> Logical Operator/2
  VfMDCC_UdVal_V/1 -> Do_Inverse_Park_Transform/1(VfMDCC_UdVal_V)
  VfMDCC_UqVal_V/1 -> Do_Inverse_Park_Transform/2(VfMDCC_UqVal_V)
  VfMDCC_SinEAngleNextPWMValue_NULL/1 -> Do_Inverse_Park_Transform/3(VfMDCC_SinEAngleNextPWMValue_NULL)
  VfMDCC_CosEAngleNextPWMValue_NULL/1 -> Do_Inverse_Park_Transform/4(VfMDCC_CosEAngleNextPWMValue_NULL)

== system MDCC/DoCurCtr_sys/MDCC/UdUqCalc_Sys/MDCC_Inverse_Park_rotation_coef_cp ==
  VuMDCC_MotorPositionCnt_NULL : Inport
  VuMDTM_PwmFrequency_Hz : Inport  Port=2
  VfMDSP_MotorMSpeed_rads : Inport  Port=3
  Add : Sum
  Constant : Constant  Value=GLBCal_Ke_MotorPolePairsNum_NULL
  Constant1 : Constant  Value=2^KuMDCC_PositionResolution_NULL  VectorParams1D=off
  Constant3 : Constant  Value=single(1/(2*pi))
  Cos12bit : LookupNDDirect  NumberOfTableDimensions=1  Table=CosTable12bit_Y  TableDataTypeStr=single
  Data Type Conversion : DataTypeConversion  OutDataTypeStr=uint16
  Divide : Product  Inputs=*/
  KfMDCC_InvParkCpPeriodTimesT_NULL : Constant  Value=KfMDCC_InvParkCpPeriodTimesT_NULL
  Math Function : Math  Operator=mod  SignedPower=on  SaturateOnIntegerOverflow=on
  Product : Product  Inputs=3
  Product1 : Product
  Product2 : Product
  Sin12bit : LookupNDDirect  NumberOfTableDimensions=1  Table=SinTable12bit_Y  TableDataTypeStr=single
  VfMDCC_SinEAngleNextPWMValue_NULL : Outport
  VfMDCC_CosEAngleNextPWMValue_NULL : Outport  Port=2
  wires:
  Sin12bit/1 -> VfMDCC_SinEAngleNextPWMValue_NULL/1
  VuMDTM_PwmFrequency_Hz/1 -> Divide/2
  Constant/1 -> Product/2
  Product/1 -> Divide/1
  Product1/1 -> Add/2  "VfMDCC_PositionCpVal_NULL"
  Math Function/1 -> Cos12bit/1, Sin12bit/1
  Add/1 -> Data Type Conversion/1
  Constant1/1 -> Product1/2, Math Function/2
  Data Type Conversion/1 -> Math Function/1
  VfMDSP_MotorMSpeed_rads/1 -> Product/1
  Constant3/1 -> Product/3
  VuMDCC_MotorPositionCnt_NULL/1 -> Add/1
  Cos12bit/1 -> VfMDCC_CosEAngleNextPWMValue_NULL/1
  Divide/1 -> Product2/1
  Product2/1 -> Product1/1
  KfMDCC_InvParkCpPeriodTimesT_NULL/1 -> Product2/2

== system MDCC/DoCurCtr_sys/MDCC/UdUqCalc_Sys/MDCC_MCF_Sys ==
  VfMDSP_PhaseUCurVal_A : Inport
  VfMDSP_PhaseVCurVal_A : Inport  Port=2
  VfMDSP_PhaseWCurVal_A : Inport  Port=3
  VuMDTM_PwmFrequency_Hz : Inport  Port=4
  VfMDSP_MotorESpeed_rads : Inport  Port=5
  VuMDCC_MotorPositionCnt_NULL : Inport  Port=6  OutMin=[0]  OutMax=[4095]
  VfMDTL_TorqueCmd_Nm : Inport  Port=7
  VfMDSP_DCLinkVolVal_V : Inport  Port=8
  Bus Creator : BusCreator  Inputs=2
  Bus Creator1 : BusCreator  Inputs=2
  Bus Selector : BusSelector  OutputSignals=MCF_uAlphaHarm,MCF_uBetaHarm
  CAL_MCF_flgHarmInject_b : Constant  Value=KbMDCC_MCF_flgHarmInject_flg
  Clarke1 : Subsystem  RTWFcnName=vPwm_MDCC_Clarke  RTWFileName=MDCC
      settings: RTWSystemCode=Nonreusable function  RTWFcnNameOpts=User specified
  Constant : Constant  OutDataTypeStr=single
  Constant1 : Constant  Value=-KfMDCC_MCF_HarmInUAlphaMax_V
  Constant2 : Constant  Value=-KfMDCC_MCF_HarmInUbetaMax_V
  Constant3 : Constant  Value=KfMDCC_MCF_HarmInUAlphaMax_V
  Constant4 : Constant  Value=KfMDCC_MCF_HarmInUbetaMax_V
  Divide : Product  Inputs=*/  OutDataTypeStr=single
  Enabled Subsystem : Subsystem  TreatAsAtomicUnit=on
  Saturation : simulink/Discontinuities/Saturation Dynamic  OutMin=[]  OutMax=[]  OutDataTypeStr=Inherit: Same as second input  OutDataType=fixdt(1, 16)  OutScaling=2^-10  DoSatur=off
  Saturation1 : simulink/Discontinuities/Saturation Dynamic  OutMin=[]  OutMax=[]  OutDataTypeStr=Inherit: Same as second input  OutDataType=fixdt(1, 16)  OutScaling=2^-10  DoSatur=off
  Subsystem : Subsystem
  Switch : Switch  Criteria=u2 ~= 0
  Zero : Constant  Value=0  OutDataTypeStr=single
  Zero1 : Constant  Value=0  OutDataTypeStr=single
  MCF_uAlphaHarm : Outport  VectorParamsAs1DForOutWhenUnconnected=off
  MCF_uBetaHarm : Outport  Port=2  VectorParamsAs1DForOutWhenUnconnected=off
  wires:
  CAL_MCF_flgHarmInject_b/1 -> Switch/2, Enabled Subsystem/Enable
  Subsystem/2(VfMDCC_PhaseVCurHarmonic_A) -> Clarke1/2(VfMDCC_PhaseVCurHarmonic_A)
  Subsystem/1(VfMDCC_PhaseUCurHarmonic_A) -> Clarke1/1(VfMDCC_PhaseUCurHarmonic_A)
  VfMDSP_PhaseUCurVal_A/1 -> Subsystem/1(VfMDSP_PhaseUCurVal_A)
  Constant2/1 -> Saturation1/3
  Clarke1/1(VfMDCC_AlphaCurHarmonic_A) -> Enabled Subsystem/1(VfMDCC_AlphaCurHarmonic_A)
  Constant1/1 -> Saturation/3
  Subsystem/3(VfMDCC_PhaseWCurHarmonic_A) -> Clarke1/3(VfMDCC_PhaseWCurHarmonic_A)
  VfMDSP_DCLinkVolVal_V/1 -> Enabled Subsystem/7(MCF_uDcLnk)
  VfMDSP_MotorESpeed_rads/1 -> Subsystem/5(VfMDSP_MotorESpeed_rads), Enabled Subsystem/6(VfMDSP_MotorESpeed_rads)
  Clarke1/2(VfMDCC_BetaCurHarmonic_A) -> Enabled Subsystem/3(VfMDCC_BetaCurHarmonic_A)
  Constant/1 -> Divide/1
  Divide/1 -> Enabled Subsystem/5(VfMDTM_PwmCycleTime_s), Subsystem/4(VfMDTM_PwmCycleTime_s)
  VuMDCC_MotorPositionCnt_NULL/1 -> Enabled Subsystem/2(VuMDCC_MotorPositionCnt_NULL)
  VfMDSP_PhaseVCurVal_A/1 -> Subsystem/2(VfMDSP_PhaseVCurVal_A)
  Constant3/1 -> Saturation/1
  VfMDTL_TorqueCmd_Nm/1 -> Enabled Subsystem/4(VfMDTL_TorqueCmd_Nm)
  VuMDTM_PwmFrequency_Hz/1 -> Divide/2
  Zero/1 -> Bus Creator1/1  "MCF_uAlphaHarm"
  Bus Selector/2 -> Saturation1/2  "<MCF_uBetaHarm>"
  VfMDSP_PhaseWCurVal_A/1 -> Subsystem/3(VfMDSP_PhaseWCurVal_A)
  Enabled Subsystem/1(MCF_uAlphaHarm) -> Bus Creator/1  "MCF_uAlphaHarm"
  Switch/1 -> Bus Selector/1
  Zero1/1 -> Bus Creator1/2  "MCF_uBetaHarm"
  Saturation/1 -> MCF_uAlphaHarm/1
  Saturation1/1 -> MCF_uBetaHarm/1
  Bus Creator1/1 -> Switch/3
  Bus Creator/1 -> Switch/1
  Bus Selector/1 -> Saturation/2  "<MCF_uAlphaHarm>"
  Constant4/1 -> Saturation1/1
  Enabled Subsystem/2(MCF_uBetaHarm) -> Bus Creator/2  "MCF_uBetaHarm"

== system MDCC/DoCurCtr_sys/MDCC/UdUqCalc_Sys/ModDegPwrFacCal ==
  VfMDCC_UdVal_V : Inport
  VfMDCC_UqVal_V : Inport  Port=2
  VfMDCC_DCLinkVolUsed_V : Inport  Port=3
  VfMDCC_dCur_A : Inport  Port=4
  VfMDCC_qCur_A : Inport  Port=5
  Divide : Product  Inputs=/*/
  Divide1 : Product  Inputs=*/
  Divide2 : Product  Inputs=*/
  Gain : Gain  Gain=1.732  OutDataTypeStr=single
  Gain1 : Gain  Gain=3/sqrt(6)
  Terminator : Terminator
  Terminator1 : Terminator
  isCal : Subsystem
  pwrCal : Subsystem
  usCal : Subsystem
  VfMDCC_DCLinkCurVal_A : Outport
  wires:
  VfMDCC_UdVal_V/1 -> pwrCal/3(ud), usCal/1(ud)
  VfMDCC_UqVal_V/1 -> pwrCal/4(uq), usCal/2(uq)
  VfMDCC_dCur_A/1 -> pwrCal/1(id), isCal/1(id)
  VfMDCC_qCur_A/1 -> pwrCal/2(iq), isCal/2(iq)
  pwrCal/1(pwr) -> Divide/2, Gain1/1
  isCal/1(is) -> Divide/1
  usCal/1(us) -> Gain/1, Divide/3
  Divide/1 -> Terminator/1  "MDCC_VfMDCC_PwrFac_NULL"
  Gain/1 -> Divide1/1
  VfMDCC_DCLinkVolUsed_V/1 -> Divide2/2, Divide1/2
  Divide1/1 -> Terminator1/1  "VfMDCC_ModDeg_NULL"
  Gain1/1 -> Divide2/1
  Divide2/1 -> VfMDCC_DCLinkCurVal_A/1

== system MDCC/DoCurCtr_sys/MDCC/UdUqCalc_Sys/Park ==
  VfMDCC_EAngleCos_NULL : Inport
  VfMDCC_EAngleSin_NULL : Inport  Port=2
  VfMDCC_AlphaCur_A : Inport  Port=3
  VfMDCC_BetaCur_A : Inport  Port=4
  Product{,1..3} (4 alike) : Product
  Subtract : Sum
  Subtract1 : Sum  Inputs=+-
  VfMDCC_dCur_A : Outport
  VfMDCC_qCur_A : Outport  Port=2
  wires:
  VfMDCC_AlphaCur_A/1 -> Product3/1, Product/1
  VfMDCC_EAngleCos_NULL/1 -> Product2/2, Product/2
  VfMDCC_BetaCur_A/1 -> Product2/1, Product1/1
  VfMDCC_EAngleSin_NULL/1 -> Product3/2, Product1/2
  Product/1 -> Subtract/1
  Product1/1 -> Subtract/2
  Subtract/1 -> VfMDCC_dCur_A/1  "VfMDCC_dCur_A"
  Product2/1 -> Subtract1/1
  Product3/1 -> Subtract1/2
  Subtract1/1 -> VfMDCC_qCur_A/1  "VfMDCC_qCur_A"

== system MDCC/DoCurCtr_sys/MDCC/UdUqCalc_Sys/SelfHeating ==
  VbMDSP_McuFSelfheatingMode_flg : Inport
  VfMDTM_SelfHeatingEAngle_NULL : Inport  Port=2
  VbMDTM_SelfHeatingSinWaveEn_flg : Inport  Port=3
  Enable : EnablePort
  Constant : Constant  Value=0  OutDataTypeStr=single
  Subsystem1 : Subsystem
  VfMDCC_SelfHeatingUdVal_V : Outport
  VfMDCC_SelfHeatingUqVal_V : Outport  Port=2
  VbMDCC_SelfHeatingStop_flg : Outport  Port=3
  wires:
  VfMDTM_SelfHeatingEAngle_NULL/1 -> Subsystem1/1(VfMDTM_SelfHeatingEAngle_NULL)
  Subsystem1/1(VfMDCC_SelfHeatingUdVal_V) -> VfMDCC_SelfHeatingUdVal_V/1
  Constant/1 -> VfMDCC_SelfHeatingUqVal_V/1
  VbMDTM_SelfHeatingSinWaveEn_flg/1 -> Subsystem1/2(VbMDTM_SelfHeatingSinWaveEn_flg)
  Subsystem1/2(VbMDCC_SelfHeatingStop_flg) -> VbMDCC_SelfHeatingStop_flg/1
  VbMDSP_McuFSelfheatingMode_flg/1 -> Subsystem1/3(VbMDSP_McuFSelfheatingMode_flg)

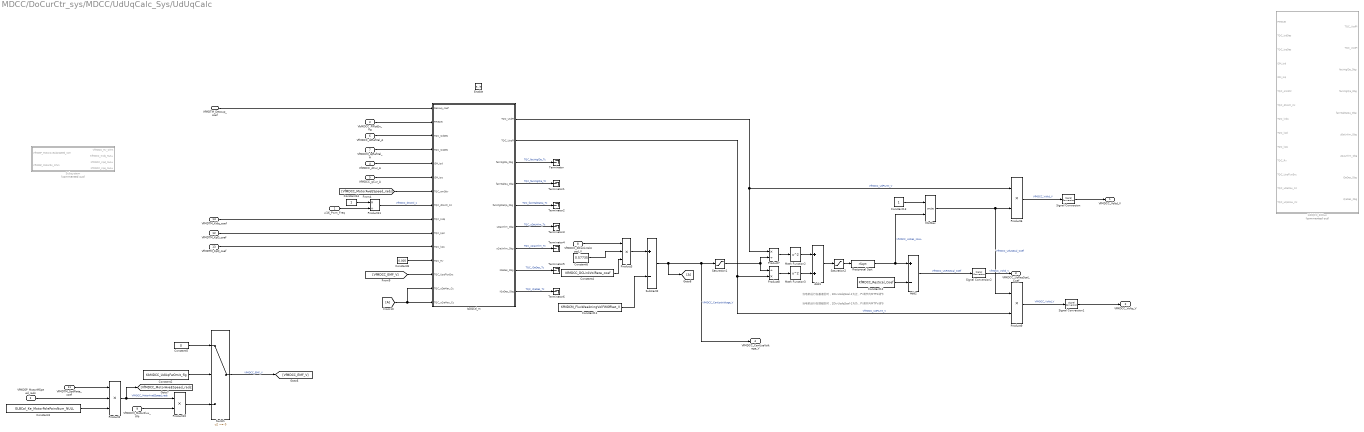
== system MDCC/DoCurCtr_sys/MDCC/UdUqCalc_Sys/UdUqCalc ==
  note: 当电机运行在基速区时，1DivUsdqScal-1为正，PI调节向MTPA调节
  note: 当电机运行在弱磁区时，1DivUsdqScal-1为负，PI调节向MTPV调节
  ui16_Pwm_Freq : Inport
  VfMDSP_MotorMSpeed_rads : Inport  Port=2
  VbMDCC_PIRstEn_flg : Inport  Port=3
  VfMDCC_dCur_A : Inport  Port=4
  VfMDCC_qCur_A : Inport  Port=5
  VfMDCC_IdRefVal_A : Inport  Port=6
  VfMDCM_IqRefVal_A : Inport  Port=7
  VfMDCC_DCLinkVolUsed_V : Inport  Port=8
  VfMDCM_MotorFlux_Wb : Inport  Port=9
  VfMDTM_Decoup_coef : Inport  Port=10
  VfMDTM_SpdRate_coef : Inport  Port=11
  VfMDTM_KpD_coef : Inport  Port=12
  VfMDTM_KpQ_coef : Inport  Port=13
  VfMDTM_Kidq_coef : Inport  Port=14
  Enable : EnablePort  StatesWhenEnabling=reset
  Add1 : Sum  OutDataTypeStr=single
  Add2 : Sum  Inputs=+-  OutDataTypeStr=single
  Constant11 : Constant  Value=KfMDCM_FluxWeakningVolFWOffset_V
  Constant12 : Constant  Value=KfMDCC_ResScal_Coef  OutDataTypeStr=Inherit: Inherit via back propagation
  Constant13 : Constant  OutDataTypeStr=Inherit: Inherit via back propagation
  Constant14 : Constant  OutDataTypeStr=Inherit: Inherit via back propagation
  Constant2 : Constant  Value=KbMDCC_UdUqFwOmit_flg
  Constant3 : Constant  Value=GLBCal_Ke_MotorPolePairsNum_NULL
  Constant4 : Constant  Value=KfMDCC_DCLinkVolRate_coef
  Constant5 : Constant  Value=0  OutDataTypeStr=Inherit: Inherit via back propagation
  Constant6 : Constant  Value=0.57735  OutDataTypeStr=single
  Constant8 : Constant  Value=0.005  OutDataTypeStr=Inherit: Inherit via back propagation
  IsDQCtl_200us : Subsystem  Commented=on  Variant=on  VariantControlMode=label  VariantControl=Choice  LabelModeActiveChoice=IsDQCtl_m
  IsDQCtl_m : MATLAB Function  TreatAsAtomicUnit=on  VariantControl=IsDQCtl_m
      settings: RTWSystemCode=Nonreusable function  RTWFcnNameOpts=Use subsystem name
  Math Function2 : Math  Operator=square  SignedPower=on  SaturateOnIntegerOverflow=on
  Math Function3 : Math  Operator=square  SignedPower=on  SaturateOnIntegerOverflow=on
  MinMax : MinMax  Inputs=2
  Product10 : Product  OutDataTypeStr=single  RndMeth=Round
  Product11 : Product  Inputs=*/  OutDataTypeStr=single
  Product2 : Product  Inputs=3  OutDataTypeStr=single  RndMeth=Round
  Product3 : Product  Inputs=3
  Product6 : Product
  Product7 : Product  Inputs=*/
  Product8 : Product  Inputs=/*
  Product9 : Product
  Reciprocal Sqrt : Sqrt  Operator=rSqrt  SaturateOnIntegerOverflow=on
  Saturation1 : Saturate  UpperLimit=100000  LowerLimit=0.000001
  Saturation2 : Saturate  UpperLimit=100000  LowerLimit=0.000001
  Signal Conversion : SignalConversion  OverrideOpt=off
  Signal Conversion1 : SignalConversion  OverrideOpt=off
  Signal Conversion2 : SignalConversion  OverrideOpt=off
  Subsystem : Subsystem  Commented=on
  Subtract2 : Sum  Inputs=+-
  Switch : Switch  Criteria=u2 ~= 0
  Terminator{,1..6} (7 alike) : Terminator
  VfMDCC_Voltd_V : Outport
  VfMDCC_Voltq_V : Outport  Port=2
  VfMDCC_UsResScal_Coef : Outport  Port=3
  VfMDCC_CanUseVoltage_V : Outport  Port=4
  wires:
  Signal Conversion/1 -> VfMDCC_Voltd_V/1
  Signal Conversion1/1 -> VfMDCC_Voltq_V/1
  Constant2/1 -> Switch/2
  Constant5/1 -> Switch/1
  Product2/1 -> [VfMDCC_MotorAveESpeed_rads], Product10/1  "VfMDCC_MotorAveESpeed_rads"
  VfMDSP_MotorMSpeed_rads/1 -> Product2/2
  VfMDCM_MotorFlux_Wb/1 -> Product10/2
  Constant3/1 -> Product2/3
  Switch/1 -> [VfMDCC_EMF_V]  "VfMDCC_EMF_V"
  Product6/1 -> Signal Conversion/1  "VfMDCC_Voltd_V"
  MinMax/1 -> Product6/2, Product9/1  "VfMDCC_UdUqScal_Coef"
  Product9/1 -> Signal Conversion1/1  "VfMDCC_Voltd_V"
  Product7/1 -> Math Function2/1
  VfMDCC_DCLinkVolUsed_V/1 -> Product3/1
  Add1/1 -> Saturation2/1
  Constant6/1 -> Product3/2
  Product8/1 -> Math Function3/1
  Constant13/1 -> MinMax/1
  Constant11/1 -> Subtract2/2
  Product3/1 -> Subtract2/1
  Saturation2/1 -> Reciprocal Sqrt/1
  Reciprocal Sqrt/1 -> Add2/1, MinMax/2  "VfMDCC_UsRes_NULL"
  Math Function2/1 -> Add1/1
  Add2/1 -> Signal Conversion2/1  "VfMDCC_UsResScal_Coef"
  Math Function3/1 -> Add1/2
  Subtract2/1 -> [A], Saturation1/1, VfMDCC_CanUseVoltage_V/1  "VfMDCC_CanUseVoltage_V"
  Saturation1/1 -> Product7/2, Product8/1
  Constant12/1 -> Add2/2
  Product10/1 -> Switch/3
  ui16_Pwm_Freq/1 -> Product11/2
  Constant14/1 -> Product11/1
  VbMDCC_PIRstEn_flg/1 -> IsDQCtl_m/2(PIReset)
  VfMDCC_IdRefVal_A/1 -> IsDQCtl_m/3(TQC_IsdDes)
  VfMDCM_IqRefVal_A/1 -> IsDQCtl_m/4(TQC_IsqDes)
  VfMDCC_dCur_A/1 -> IsDQCtl_m/5(ISM_Isd)
  VfMDCC_qCur_A/1 -> IsDQCtl_m/6(ISM_Isq)
  [VfMDCC_MotorAveESpeed_rads] -> IsDQCtl_m/7(TQC_omSttr)
  Product11/1 -> IsDQCtl_m/8(TQC_dtIsctl_Cc)  "VfMDCC_dtIsCtl_s"
  VfMDTM_Kidq_coef/1 -> IsDQCtl_m/9(TQC_kidq)
  VfMDTM_KpD_coef/1 -> IsDQCtl_m/10(TQC_kpd)
  VfMDTM_KpQ_coef/1 -> IsDQCtl_m/11(TQC_kpq)
  Constant8/1 -> IsDQCtl_m/12(TQC_Rv)
  [VfMDCC_EMF_V] -> IsDQCtl_m/13(TQC_UsqFluxExc)
  IsDQCtl_m/1(TQC_UsdPI) -> Product7/1, Product6/1  "VfMDCC_UdPILmt_V"
  IsDQCtl_m/2(TQC_UsqPI) -> Product9/2, Product8/2  "VfMDCC_UqPILmt_V"
  IsDQCtl_m/3(facIntglDa_Dbg) -> Terminator/1  "TQC_facIntglDa_Tc"
  IsDQCtl_m/4(facIntglQa_Dbg) -> Terminator1/1  "TQC_facIntglQa_Tc"
  IsDQCtl_m/5(facIntglDaQa_Dbg) -> Terminator2/1  "TQC_facIntglDaQa_Tc"
  IsDQCtl_m/6(uDaUnlim_Dbg) -> Terminator3/1  "TQC_uDaUnlim_Tc"
  IsDQCtl_m/7(uQaUnlim_Dbg) -> Terminator4/1  "TQC_uQaUnlim_Tc"
  IsDQCtl_m/8(iDaDes_Dbg) -> Terminator5/1  "TQC_iDaDes_Tc"
  IsDQCtl_m/9(iQaDes_Dbg) -> Terminator6/1  "TQC_iQaDes_Tc"
  Constant4/1 -> Product3/3
  [A] -> IsDQCtl_m/14(TQC_uDaMax_Cc), IsDQCtl_m/15(TQC_uQaMax_Cc)
  VfMDTM_Decoup_coef/1 -> IsDQCtl_m/1(Decoup_coef)
  VfMDTM_SpdRate_coef/1 -> Product2/1
  Signal Conversion2/1 -> VfMDCC_UsResScal_Coef/1  "VfMDCC_Voltd_V"

== system MDCC/DoCurCtr_sys/MDCC/UdUqCalc_Sys/UdUqSet ==
  Enable : EnablePort  StatesWhenEnabling=reset
  Constant : Constant  Value=KfMDCC_DebugUdCmd_V
  Constant1 : Constant  Value=KfMDCC_DebugUqCmd_V
  VfMDCC_UdVal_V : Outport
  VfMDCC_UqVal_V : Outport  Port=2
  wires:
  Constant/1 -> VfMDCC_UdVal_V/1
  Constant1/1 -> VfMDCC_UqVal_V/1

== system MDCC/DoCurCtr_sys/MDCC/IrmsCalc_Sys/Subsystem3/Subsystem ==
  Earliest_Element : Inport
  Element_Inlet : Inport  Port=2
  Add : Sum  Inputs=+-
  Add1 : Sum
  Delay : Delay  DelayLength=1
  Rms : Outport
  wires:
  Add1/1 -> Rms/1, Delay/1
  Earliest_Element/1 -> Add/2
  Element_Inlet/1 -> Add/1
  Add/1 -> Add1/1
  Delay/1 -> Add1/2

== system MDCC/DoCurCtr_sys/MDCC/IrmsCalc_Sys/Subsystem3/Subsystem1 ==
  Earliest_Element : Inport
  Element_Inlet : Inport  Port=2
  Add : Sum  Inputs=+-
  Add1 : Sum
  Delay : Delay  DelayLength=1
  Rms : Outport
  wires:
  Add1/1 -> Rms/1, Delay/1
  Earliest_Element/1 -> Add/2
  Element_Inlet/1 -> Add/1
  Add/1 -> Add1/1
  Delay/1 -> Add1/2

== system MDCC/DoCurCtr_sys/MDCC/IrmsCalc_Sys/Subsystem3/Subsystem2 ==
  Earliest_Element : Inport
  Element_Inlet : Inport  Port=2
  Add : Sum  Inputs=+-
  Add1 : Sum
  Delay : Delay  DelayLength=1
  Rms : Outport
  wires:
  Add1/1 -> Rms/1, Delay/1
  Earliest_Element/1 -> Add/2
  Element_Inlet/1 -> Add/1
  Add/1 -> Add1/1
  Delay/1 -> Add1/2

== system MDCC/DoCurCtr_sys/MDCC/SVM_Calc/DeadComp_Sys/DeadCur_Calc ==
  IsdDes_A : Inport
  IsqDes_A : Inport  Port=2
  IsdFb_A : Inport  Port=3
  IsqFb_A : Inport  Port=4
  FrqRtrEl_Hz : Inport  Port=5
  agPreRtrEl : Inport  Port=6
  PwmFreq_Hz : Inport  Port=7
  Gain : Gain  Gain=6*pi
  Inverse_Clarke_Transform : Subsystem  TreatAsAtomicUnit=on
      settings: RTWSystemCode=Nonreusable function  RTWFcnNameOpts=Use subsystem name
  IsdqSelect_Calc : Subsystem  TreatAsAtomicUnit=on
      settings: RTWSystemCode=Nonreusable function  RTWFcnNameOpts=Use subsystem name
  N_Select_Calc : Subsystem  TreatAsAtomicUnit=on
      settings: RTWSystemCode=Nonreusable function  RTWFcnNameOpts=Use subsystem name
  Signal Copy : SignalConversion  OverrideOpt=off
  Signal Copy1 : SignalConversion  OverrideOpt=off
  SineCosineLookup_Calc : Subsystem  TreatAsAtomicUnit=on
      settings: RTWSystemCode=Nonreusable function  RTWFcnNameOpts=Use subsystem name
  iPark_Calc : Subsystem  TreatAsAtomicUnit=on
      settings: RTWSystemCode=Nonreusable function  RTWFcnNameOpts=Use subsystem name
  iaPre : Outport
  ibPre : Outport  Port=2
  icPre : Outport  Port=3
  CntSctrIs : Outport  Port=4
  wires:
  iPark_Calc/1(Alpha) -> Signal Copy/1
  IsdqSelect_Calc/2(Isq_A) -> iPark_Calc/2(Qs), N_Select_Calc/5(Isq_A)
  IsdDes_A/1 -> IsdqSelect_Calc/1(IsdDes_A)
  IsdqSelect_Calc/1(Isd_A) -> iPark_Calc/1(Ds), N_Select_Calc/4(Isd_A)
  SineCosineLookup_Calc/2(cos) -> iPark_Calc/4(cos)
  Inverse_Clarke_Transform/2(b) -> ibPre/1
  SineCosineLookup_Calc/1(sin) -> iPark_Calc/3(sin)
  IsqFb_A/1 -> IsdqSelect_Calc/4(IsqFb_A)
  Inverse_Clarke_Transform/3(c) -> icPre/1
  iPark_Calc/2(Beta) -> Signal Copy1/1
  IsdFb_A/1 -> IsdqSelect_Calc/3(IsdFb_A)
  FrqRtrEl_Hz/1 -> Gain/1
  IsqDes_A/1 -> IsdqSelect_Calc/2(IsqDes_A)
  agPreRtrEl/1 -> N_Select_Calc/2(eMtrPos_NULL)
  Inverse_Clarke_Transform/1(a) -> iaPre/1
  PwmFreq_Hz/1 -> N_Select_Calc/3(VfPwmFreq_Hz)
  Gain/1 -> N_Select_Calc/1(eMtrSpd_rads)
  N_Select_Calc/2(Select_N) -> CntSctrIs/1
  N_Select_Calc/1(PreMtrPos) -> SineCosineLookup_Calc/1(PreMtrPos)
  Signal Copy/1 -> Inverse_Clarke_Transform/1(Alpha)
  Signal Copy1/1 -> Inverse_Clarke_Transform/2(Beta)
